simulink model "Experiment1_model"  (R2022a)
settings: Solver=FixedStepAuto  StartTime=0.0  StopTime=20  RelTol=1e-3
libraries: slpidlib x32, slctrlblks x18
(part 3 of 5)

== system Experiment1_model/Controller3 PID/controller robot7 ==
  x_rob2 : Inport
  Add : Sum
  Demux : Demux  Outputs=2
  Demux1 : Demux  Outputs=2
  Mux : Mux  Inputs=2
  PID Controller : slpidlib/PID Controller  Controller=PID  Form=Parallel  TimeDomain=Continuous-time  UseExternalTs=off  SampleTime=-1  IntegratorMethod=Forward Euler  FilterMethod=Forward Euler  ControllerParametersSource=internal  P=5  I=0  UseKiTs=off  D=0  N=100  UseFilter=on  TunerSelectOption=Transfer Function Based (PID Tuner App)  InitialConditionSource=internal  InitialConditionForIntegrator=0  InitialConditionForFilter=0  DifferentiatorICPrevScaledInput=0  ExternalReset=none  TrackingMode=off  Kt=1  LimitOutput=off  SatLimitsSource=internal  UpperSaturationLimit=inf  LowerSaturationLimit=-inf  LinearizeAsGain=on  AntiWindupMode=none  Kb=1  POutMin=[]  POutMax=[]  IOutMin=[]  IOutMax=[]  DOutMin=[]  DOutMax=[]  NOutMin=[]  NOutMax=[]  SumOutMin=[]  SumOutMax=[]  SaturationOutMin=[]  SaturationOutMax=[]  PParamMin=[]  PParamMax=[]  IParamMin=[]  IParamMax=[]  DParamMin=[]  DParamMax=[]  NParamMin=[]  NParamMax=[]  KbParamMin=[]  KbParamMax=[]  KtParamMin=[]  KtParamMax=[]  KbOutMin=[]  KbOutMax=[]  KtOutMin=[]  KtOutMax=[]  IntegratorOutMin=[]  IntegratorOutMax=[]  FilterOutMin=[]  FilterOutMax=[]  SumI1OutMin=[]  SumI1OutMax=[]  SumI2OutMin=[]  SumI2OutMax=[]  SumI3OutMin=[]  SumI3OutMax=[]  SumI4OutMin=[]  SumI4OutMax=[]  SumDOutMin=[]  SumDOutMax=[]  DifferentiatorOutMin=[]  DifferentiatorOutMax=[]  FilterDiffOutCoefMin=[]  FilterDiffOutCoefMax=[]  ReciprocalOutMin=[]  ReciprocalOutMax=[]  SumDenOutMin=[]  SumDenOutMax=[]  SumNumOutMin=[]  SumNumOutMax=[]  DivideOutMin=[]  DivideOutMax=[]  UdiffTsProdOutMin=[]  UdiffTsProdOutMax=[]  NTsProdOutMin=[]  NTsProdOutMax=[]  UintegralTsProdOutMin=[]  UintegralTsProdOutMax=[]  UngainTsProdOutMin=[]  UngainTsProdOutMax=[]  IntegratorContinuousStateAttributes=''  IntegratorStateMustResolveToSignalObject=off  IntegratorRTWStateStorageClass=Auto  FilterContinuousStateAttributes=''  FilterStateMustResolveToSignalObject=off  FilterRTWStateStorageClass=Auto  ParallelPVariant=InternalParameters  IdealPVariant=Disabled  IVariant=InternalParameters  DVariant=InternalParameters  IntegratorVariant=Continuous  SatVariant=Disabled  AWVariant=Passthrough  PCopyVariant=Disabled  TRVariant=Disabled  FdbkBlocksVariant=Forward  IdealPFdbkVariant=Disabled  SatFdbkVariant=Disabled  DerivativeFilterVariant=ContFilter  NVariant=InternalParameters  NCopyVariant=Disabled  FilterICVariant=InternalICsFilter  IntegratorICVariant=InternalICs  ExternalResetVariant=Disabled  TRSumVariant=Passthrough  SumFdbkVariant=Disabled  SumVariant=Sum_PID  TsampFilterVariant=InternalTs  TsampNgainVariant=Passthrough  TsampIntegralVariant=Passthrough  ExternalSaturationOutDataTypeStr=Inherit: Same as second input  aMode=0
  Ref_p1 : Constant  Value=[-10;10]  VectorParams1D=off
  Ref_v1 : Constant  Value=[0;0]  VectorParams1D=off
  Sum : Sum  Inputs=+-|
  Sum1 : Sum  Inputs=|-+
  u07 : Outport
  wires:
  x_rob2/1 -> Demux/1
  Demux/1 -> Sum/2
  Ref_p1/1 -> Sum/1
  Demux/2 -> Sum1/1
  Ref_v1/1 -> Sum1/2
  PID Controller/1 -> Demux1/1
  Demux1/2 -> Add/2
  Add/1 -> u07/1
  Demux1/1 -> Add/1
  Mux/1 -> PID Controller/1
  Sum1/1 -> Mux/2
  Sum/1 -> Mux/1

== system Experiment1_model/Controller3 PID/controller robot8 ==
  x_rob2 : Inport
  Add : Sum
  Demux : Demux  Outputs=2
  Demux1 : Demux  Outputs=2
  Mux : Mux  Inputs=2
  PID Controller : slpidlib/PID Controller  Controller=PID  Form=Parallel  TimeDomain=Continuous-time  UseExternalTs=off  SampleTime=-1  IntegratorMethod=Forward Euler  FilterMethod=Forward Euler  ControllerParametersSource=internal  P=5  I=0  UseKiTs=off  D=0  N=100  UseFilter=on  TunerSelectOption=Transfer Function Based (PID Tuner App)  InitialConditionSource=internal  InitialConditionForIntegrator=0  InitialConditionForFilter=0  DifferentiatorICPrevScaledInput=0  ExternalReset=none  TrackingMode=off  Kt=1  LimitOutput=off  SatLimitsSource=internal  UpperSaturationLimit=inf  LowerSaturationLimit=-inf  LinearizeAsGain=on  AntiWindupMode=none  Kb=1  POutMin=[]  POutMax=[]  IOutMin=[]  IOutMax=[]  DOutMin=[]  DOutMax=[]  NOutMin=[]  NOutMax=[]  SumOutMin=[]  SumOutMax=[]  SaturationOutMin=[]  SaturationOutMax=[]  PParamMin=[]  PParamMax=[]  IParamMin=[]  IParamMax=[]  DParamMin=[]  DParamMax=[]  NParamMin=[]  NParamMax=[]  KbParamMin=[]  KbParamMax=[]  KtParamMin=[]  KtParamMax=[]  KbOutMin=[]  KbOutMax=[]  KtOutMin=[]  KtOutMax=[]  IntegratorOutMin=[]  IntegratorOutMax=[]  FilterOutMin=[]  FilterOutMax=[]  SumI1OutMin=[]  SumI1OutMax=[]  SumI2OutMin=[]  SumI2OutMax=[]  SumI3OutMin=[]  SumI3OutMax=[]  SumI4OutMin=[]  SumI4OutMax=[]  SumDOutMin=[]  SumDOutMax=[]  DifferentiatorOutMin=[]  DifferentiatorOutMax=[]  FilterDiffOutCoefMin=[]  FilterDiffOutCoefMax=[]  ReciprocalOutMin=[]  ReciprocalOutMax=[]  SumDenOutMin=[]  SumDenOutMax=[]  SumNumOutMin=[]  SumNumOutMax=[]  DivideOutMin=[]  DivideOutMax=[]  UdiffTsProdOutMin=[]  UdiffTsProdOutMax=[]  NTsProdOutMin=[]  NTsProdOutMax=[]  UintegralTsProdOutMin=[]  UintegralTsProdOutMax=[]  UngainTsProdOutMin=[]  UngainTsProdOutMax=[]  IntegratorContinuousStateAttributes=''  IntegratorStateMustResolveToSignalObject=off  IntegratorRTWStateStorageClass=Auto  FilterContinuousStateAttributes=''  FilterStateMustResolveToSignalObject=off  FilterRTWStateStorageClass=Auto  ParallelPVariant=InternalParameters  IdealPVariant=Disabled  IVariant=InternalParameters  DVariant=InternalParameters  IntegratorVariant=Continuous  SatVariant=Disabled  AWVariant=Passthrough  PCopyVariant=Disabled  TRVariant=Disabled  FdbkBlocksVariant=Forward  IdealPFdbkVariant=Disabled  SatFdbkVariant=Disabled  DerivativeFilterVariant=ContFilter  NVariant=InternalParameters  NCopyVariant=Disabled  FilterICVariant=InternalICsFilter  IntegratorICVariant=InternalICs  ExternalResetVariant=Disabled  TRSumVariant=Passthrough  SumFdbkVariant=Disabled  SumVariant=Sum_PID  TsampFilterVariant=InternalTs  TsampNgainVariant=Passthrough  TsampIntegralVariant=Passthrough  ExternalSaturationOutDataTypeStr=Inherit: Same as second input  aMode=0
  Ref_p1 : Constant  Value=[-10;0.5]  VectorParams1D=off
  Ref_v1 : Constant  Value=[0;0]  VectorParams1D=off
  Sum : Sum  Inputs=+-|
  Sum1 : Sum  Inputs=|-+
  u08 : Outport
  wires:
  x_rob2/1 -> Demux/1
  Demux/1 -> Sum/2
  Ref_p1/1 -> Sum/1
  Demux/2 -> Sum1/1
  Ref_v1/1 -> Sum1/2
  PID Controller/1 -> Demux1/1
  Demux1/2 -> Add/2
  Add/1 -> u08/1
  Demux1/1 -> Add/1
  Mux/1 -> PID Controller/1
  Sum1/1 -> Mux/2
  Sum/1 -> Mux/1

== system Experiment1_model/Controller3 PID1/controller robot1 ==
  x_rob1 : Inport
  Add : Sum
  Demux : Demux  Outputs=2
  Demux1 : Demux  Outputs=2
  Demux2 : Demux  Outputs=2
  Mux : Mux  Inputs=2
  PID Controller : slpidlib/PID Controller  Controller=PID  Form=Parallel  TimeDomain=Continuous-time  UseExternalTs=off  SampleTime=-1  IntegratorMethod=Forward Euler  FilterMethod=Forward Euler  ControllerParametersSource=internal  P=5  I=0.0000001  UseKiTs=off  D=0.01  N=1  UseFilter=on  TunerSelectOption=Transfer Function Based (PID Tuner App)  InitialConditionSource=internal  InitialConditionForIntegrator=0  InitialConditionForFilter=0  DifferentiatorICPrevScaledInput=0  ExternalReset=none  TrackingMode=off  Kt=1  LimitOutput=off  SatLimitsSource=internal  UpperSaturationLimit=inf  LowerSaturationLimit=-inf  LinearizeAsGain=on  AntiWindupMode=none  Kb=1  POutMin=[]  POutMax=[]  IOutMin=[]  IOutMax=[]  DOutMin=[]  DOutMax=[]  NOutMin=[]  NOutMax=[]  SumOutMin=[]  SumOutMax=[]  SaturationOutMin=[]  SaturationOutMax=[]  PParamMin=[]  PParamMax=[]  IParamMin=[]  IParamMax=[]  DParamMin=[]  DParamMax=[]  NParamMin=[]  NParamMax=[]  KbParamMin=[]  KbParamMax=[]  KtParamMin=[]  KtParamMax=[]  KbOutMin=[]  KbOutMax=[]  KtOutMin=[]  KtOutMax=[]  IntegratorOutMin=[]  IntegratorOutMax=[]  FilterOutMin=[]  FilterOutMax=[]  SumI1OutMin=[]  SumI1OutMax=[]  SumI2OutMin=[]  SumI2OutMax=[]  SumI3OutMin=[]  SumI3OutMax=[]  SumI4OutMin=[]  SumI4OutMax=[]  SumDOutMin=[]  SumDOutMax=[]  DifferentiatorOutMin=[]  DifferentiatorOutMax=[]  FilterDiffOutCoefMin=[]  FilterDiffOutCoefMax=[]  ReciprocalOutMin=[]  ReciprocalOutMax=[]  SumDenOutMin=[]  SumDenOutMax=[]  SumNumOutMin=[]  SumNumOutMax=[]  DivideOutMin=[]  DivideOutMax=[]  UdiffTsProdOutMin=[]  UdiffTsProdOutMax=[]  NTsProdOutMin=[]  NTsProdOutMax=[]  UintegralTsProdOutMin=[]  UintegralTsProdOutMax=[]  UngainTsProdOutMin=[]  UngainTsProdOutMax=[]  IntegratorContinuousStateAttributes=''  IntegratorStateMustResolveToSignalObject=off  IntegratorRTWStateStorageClass=Auto  FilterContinuousStateAttributes=''  FilterStateMustResolveToSignalObject=off  FilterRTWStateStorageClass=Auto  ParallelPVariant=InternalParameters  IdealPVariant=Disabled  IVariant=InternalParameters  DVariant=InternalParameters  IntegratorVariant=Continuous  SatVariant=Disabled  AWVariant=Passthrough  PCopyVariant=Disabled  TRVariant=Disabled  FdbkBlocksVariant=Forward  IdealPFdbkVariant=Disabled  SatFdbkVariant=Disabled  DerivativeFilterVariant=ContFilter  NVariant=InternalParameters  NCopyVariant=Disabled  FilterICVariant=InternalICsFilter  IntegratorICVariant=InternalICs  ExternalResetVariant=Disabled  TRSumVariant=Passthrough  SumFdbkVariant=Disabled  SumVariant=Sum_PID  TsampFilterVariant=InternalTs  TsampNgainVariant=Passthrough  TsampIntegralVariant=Passthrough  ExternalSaturationOutDataTypeStr=Inherit: Same as second input  aMode=0
  Ref_p1 : Constant  Value=[10;0]  VectorParams1D=off
  Ref_v1 : Constant  Value=[0;0]  VectorParams1D=off
  Scope : Scope
  Scope1 : Scope
  Sum : Sum  Inputs=+-|
  Sum1 : Sum  Inputs=|-+
  Terminator : Terminator
  u01 : Outport
  wires:
  x_rob1/1 -> Demux/1
  Demux/1 -> Sum/2
  Ref_p1/1 -> Sum/1
  Demux/2 -> Sum1/1
  Ref_v1/1 -> Sum1/2
  Sum/1 -> Mux/1, Demux2/1
  Sum1/1 -> Mux/2, Scope/1
  Mux/1 -> PID Controller/1
  PID Controller/1 -> Demux1/1
  Demux1/2 -> Add/2
  Demux1/1 -> Add/1
  Add/1 -> u01/1
  Demux2/1 -> Terminator/1
  Demux2/2 -> Scope1/1

== system Experiment1_model/Controller3 PID1/controller robot2 ==
  x_rob2 : Inport
  Add : Sum
  Demux : Demux  Outputs=2
  Demux1 : Demux  Outputs=2
  Mux : Mux  Inputs=2
  PID Controller : slpidlib/PID Controller  Controller=PID  Form=Parallel  TimeDomain=Continuous-time  UseExternalTs=off  SampleTime=-1  IntegratorMethod=Forward Euler  FilterMethod=Forward Euler  ControllerParametersSource=internal  P=5  I=0.0000001  UseKiTs=off  D=0.01  N=1  UseFilter=on  TunerSelectOption=Transfer Function Based (PID Tuner App)  InitialConditionSource=internal  InitialConditionForIntegrator=0  InitialConditionForFilter=0  DifferentiatorICPrevScaledInput=0  ExternalReset=none  TrackingMode=off  Kt=1  LimitOutput=off  SatLimitsSource=internal  UpperSaturationLimit=inf  LowerSaturationLimit=-inf  LinearizeAsGain=on  AntiWindupMode=none  Kb=1  POutMin=[]  POutMax=[]  IOutMin=[]  IOutMax=[]  DOutMin=[]  DOutMax=[]  NOutMin=[]  NOutMax=[]  SumOutMin=[]  SumOutMax=[]  SaturationOutMin=[]  SaturationOutMax=[]  PParamMin=[]  PParamMax=[]  IParamMin=[]  IParamMax=[]  DParamMin=[]  DParamMax=[]  NParamMin=[]  NParamMax=[]  KbParamMin=[]  KbParamMax=[]  KtParamMin=[]  KtParamMax=[]  KbOutMin=[]  KbOutMax=[]  KtOutMin=[]  KtOutMax=[]  IntegratorOutMin=[]  IntegratorOutMax=[]  FilterOutMin=[]  FilterOutMax=[]  SumI1OutMin=[]  SumI1OutMax=[]  SumI2OutMin=[]  SumI2OutMax=[]  SumI3OutMin=[]  SumI3OutMax=[]  SumI4OutMin=[]  SumI4OutMax=[]  SumDOutMin=[]  SumDOutMax=[]  DifferentiatorOutMin=[]  DifferentiatorOutMax=[]  FilterDiffOutCoefMin=[]  FilterDiffOutCoefMax=[]  ReciprocalOutMin=[]  ReciprocalOutMax=[]  SumDenOutMin=[]  SumDenOutMax=[]  SumNumOutMin=[]  SumNumOutMax=[]  DivideOutMin=[]  DivideOutMax=[]  UdiffTsProdOutMin=[]  UdiffTsProdOutMax=[]  NTsProdOutMin=[]  NTsProdOutMax=[]  UintegralTsProdOutMin=[]  UintegralTsProdOutMax=[]  UngainTsProdOutMin=[]  UngainTsProdOutMax=[]  IntegratorContinuousStateAttributes=''  IntegratorStateMustResolveToSignalObject=off  IntegratorRTWStateStorageClass=Auto  FilterContinuousStateAttributes=''  FilterStateMustResolveToSignalObject=off  FilterRTWStateStorageClass=Auto  ParallelPVariant=InternalParameters  IdealPVariant=Disabled  IVariant=InternalParameters  DVariant=InternalParameters  IntegratorVariant=Continuous  SatVariant=Disabled  AWVariant=Passthrough  PCopyVariant=Disabled  TRVariant=Disabled  FdbkBlocksVariant=Forward  IdealPFdbkVariant=Disabled  SatFdbkVariant=Disabled  DerivativeFilterVariant=ContFilter  NVariant=InternalParameters  NCopyVariant=Disabled  FilterICVariant=InternalICsFilter  IntegratorICVariant=InternalICs  ExternalResetVariant=Disabled  TRSumVariant=Passthrough  SumFdbkVariant=Disabled  SumVariant=Sum_PID  TsampFilterVariant=InternalTs  TsampNgainVariant=Passthrough  TsampIntegralVariant=Passthrough  ExternalSaturationOutDataTypeStr=Inherit: Same as second input  aMode=0
  Ref_p1 : Constant  Value=[8;8]  VectorParams1D=off
  Ref_v1 : Constant  Value=[0;0]  VectorParams1D=off
  Scope : Scope
  Sum : Sum  Inputs=+-|
  Sum1 : Sum  Inputs=|-+
  u02 : Outport
  wires:
  x_rob2/1 -> Demux/1
  Demux/1 -> Sum/2
  Ref_p1/1 -> Sum/1
  Demux/2 -> Sum1/1
  Ref_v1/1 -> Sum1/2
  Add/1 -> u02/1
  Demux1/2 -> Add/2
  Mux/1 -> PID Controller/1
  Sum/1 -> Scope/1, Mux/1
  Sum1/1 -> Mux/2
  PID Controller/1 -> Demux1/1
  Demux1/1 -> Add/1

== system Experiment1_model/Controller3 PID1/controller robot3 ==
  x_rob2 : Inport
  Add : Sum
  Demux : Demux  Outputs=2
  Demux1 : Demux  Outputs=2
  Mux : Mux  Inputs=2
  PID Controller : slpidlib/PID Controller  Controller=PID  Form=Parallel  TimeDomain=Continuous-time  UseExternalTs=off  SampleTime=-1  IntegratorMethod=Forward Euler  FilterMethod=Forward Euler  ControllerParametersSource=internal  P=5  I=0.0000001  UseKiTs=off  D=0.01  N=1  UseFilter=on  TunerSelectOption=Transfer Function Based (PID Tuner App)  InitialConditionSource=internal  InitialConditionForIntegrator=0  InitialConditionForFilter=0  DifferentiatorICPrevScaledInput=0  ExternalReset=none  TrackingMode=off  Kt=1  LimitOutput=off  SatLimitsSource=internal  UpperSaturationLimit=inf  LowerSaturationLimit=-inf  LinearizeAsGain=on  AntiWindupMode=none  Kb=1  POutMin=[]  POutMax=[]  IOutMin=[]  IOutMax=[]  DOutMin=[]  DOutMax=[]  NOutMin=[]  NOutMax=[]  SumOutMin=[]  SumOutMax=[]  SaturationOutMin=[]  SaturationOutMax=[]  PParamMin=[]  PParamMax=[]  IParamMin=[]  IParamMax=[]  DParamMin=[]  DParamMax=[]  NParamMin=[]  NParamMax=[]  KbParamMin=[]  KbParamMax=[]  KtParamMin=[]  KtParamMax=[]  KbOutMin=[]  KbOutMax=[]  KtOutMin=[]  KtOutMax=[]  IntegratorOutMin=[]  IntegratorOutMax=[]  FilterOutMin=[]  FilterOutMax=[]  SumI1OutMin=[]  SumI1OutMax=[]  SumI2OutMin=[]  SumI2OutMax=[]  SumI3OutMin=[]  SumI3OutMax=[]  SumI4OutMin=[]  SumI4OutMax=[]  SumDOutMin=[]  SumDOutMax=[]  DifferentiatorOutMin=[]  DifferentiatorOutMax=[]  FilterDiffOutCoefMin=[]  FilterDiffOutCoefMax=[]  ReciprocalOutMin=[]  ReciprocalOutMax=[]  SumDenOutMin=[]  SumDenOutMax=[]  SumNumOutMin=[]  SumNumOutMax=[]  DivideOutMin=[]  DivideOutMax=[]  UdiffTsProdOutMin=[]  UdiffTsProdOutMax=[]  NTsProdOutMin=[]  NTsProdOutMax=[]  UintegralTsProdOutMin=[]  UintegralTsProdOutMax=[]  UngainTsProdOutMin=[]  UngainTsProdOutMax=[]  IntegratorContinuousStateAttributes=''  IntegratorStateMustResolveToSignalObject=off  IntegratorRTWStateStorageClass=Auto  FilterContinuousStateAttributes=''  FilterStateMustResolveToSignalObject=off  FilterRTWStateStorageClass=Auto  ParallelPVariant=InternalParameters  IdealPVariant=Disabled  IVariant=InternalParameters  DVariant=InternalParameters  IntegratorVariant=Continuous  SatVariant=Disabled  AWVariant=Passthrough  PCopyVariant=Disabled  TRVariant=Disabled  FdbkBlocksVariant=Forward  IdealPFdbkVariant=Disabled  SatFdbkVariant=Disabled  DerivativeFilterVariant=ContFilter  NVariant=InternalParameters  NCopyVariant=Disabled  FilterICVariant=InternalICsFilter  IntegratorICVariant=InternalICs  ExternalResetVariant=Disabled  TRSumVariant=Passthrough  SumFdbkVariant=Disabled  SumVariant=Sum_PID  TsampFilterVariant=InternalTs  TsampNgainVariant=Passthrough  TsampIntegralVariant=Passthrough  ExternalSaturationOutDataTypeStr=Inherit: Same as second input  aMode=0
  Ref_p1 : Constant  Value=[10;-10]  VectorParams1D=off
  Ref_v1 : Constant  Value=[0;0]  VectorParams1D=off
  Sum : Sum  Inputs=+-|
  Sum1 : Sum  Inputs=|-+
  u03 : Outport
  wires:
  x_rob2/1 -> Demux/1
  Demux/1 -> Sum/2
  Ref_p1/1 -> Sum/1
  Demux/2 -> Sum1/1
  Ref_v1/1 -> Sum1/2
  Add/1 -> u03/1
  Demux1/2 -> Add/2
  Demux1/1 -> Add/1
  Sum1/1 -> Mux/2
  Sum/1 -> Mux/1
  PID Controller/1 -> Demux1/1
  Mux/1 -> PID Controller/1

== system Experiment1_model/Controller3 PID1/controller robot4 ==
  x_rob2 : Inport
  Add : Sum
  Demux : Demux  Outputs=2
  Demux1 : Demux  Outputs=2
  Mux : Mux  Inputs=2
  PID Controller : slpidlib/PID Controller  Controller=PID  Form=Parallel  TimeDomain=Continuous-time  UseExternalTs=off  SampleTime=-1  IntegratorMethod=Forward Euler  FilterMethod=Forward Euler  ControllerParametersSource=internal  P=5  I=0.0000001  UseKiTs=off  D=0.01  N=1  UseFilter=on  TunerSelectOption=Transfer Function Based (PID Tuner App)  InitialConditionSource=internal  InitialConditionForIntegrator=0  InitialConditionForFilter=0  DifferentiatorICPrevScaledInput=0  ExternalReset=none  TrackingMode=off  Kt=1  LimitOutput=off  SatLimitsSource=internal  UpperSaturationLimit=inf  LowerSaturationLimit=-inf  LinearizeAsGain=on  AntiWindupMode=none  Kb=1  POutMin=[]  POutMax=[]  IOutMin=[]  IOutMax=[]  DOutMin=[]  DOutMax=[]  NOutMin=[]  NOutMax=[]  SumOutMin=[]  SumOutMax=[]  SaturationOutMin=[]  SaturationOutMax=[]  PParamMin=[]  PParamMax=[]  IParamMin=[]  IParamMax=[]  DParamMin=[]  DParamMax=[]  NParamMin=[]  NParamMax=[]  KbParamMin=[]  KbParamMax=[]  KtParamMin=[]  KtParamMax=[]  KbOutMin=[]  KbOutMax=[]  KtOutMin=[]  KtOutMax=[]  IntegratorOutMin=[]  IntegratorOutMax=[]  FilterOutMin=[]  FilterOutMax=[]  SumI1OutMin=[]  SumI1OutMax=[]  SumI2OutMin=[]  SumI2OutMax=[]  SumI3OutMin=[]  SumI3OutMax=[]  SumI4OutMin=[]  SumI4OutMax=[]  SumDOutMin=[]  SumDOutMax=[]  DifferentiatorOutMin=[]  DifferentiatorOutMax=[]  FilterDiffOutCoefMin=[]  FilterDiffOutCoefMax=[]  ReciprocalOutMin=[]  ReciprocalOutMax=[]  SumDenOutMin=[]  SumDenOutMax=[]  SumNumOutMin=[]  SumNumOutMax=[]  DivideOutMin=[]  DivideOutMax=[]  UdiffTsProdOutMin=[]  UdiffTsProdOutMax=[]  NTsProdOutMin=[]  NTsProdOutMax=[]  UintegralTsProdOutMin=[]  UintegralTsProdOutMax=[]  UngainTsProdOutMin=[]  UngainTsProdOutMax=[]  IntegratorContinuousStateAttributes=''  IntegratorStateMustResolveToSignalObject=off  IntegratorRTWStateStorageClass=Auto  FilterContinuousStateAttributes=''  FilterStateMustResolveToSignalObject=off  FilterRTWStateStorageClass=Auto  ParallelPVariant=InternalParameters  IdealPVariant=Disabled  IVariant=InternalParameters  DVariant=InternalParameters  IntegratorVariant=Continuous  SatVariant=Disabled  AWVariant=Passthrough  PCopyVariant=Disabled  TRVariant=Disabled  FdbkBlocksVariant=Forward  IdealPFdbkVariant=Disabled  SatFdbkVariant=Disabled  DerivativeFilterVariant=ContFilter  NVariant=InternalParameters  NCopyVariant=Disabled  FilterICVariant=InternalICsFilter  IntegratorICVariant=InternalICs  ExternalResetVariant=Disabled  TRSumVariant=Passthrough  SumFdbkVariant=Disabled  SumVariant=Sum_PID  TsampFilterVariant=InternalTs  TsampNgainVariant=Passthrough  TsampIntegralVariant=Passthrough  ExternalSaturationOutDataTypeStr=Inherit: Same as second input  aMode=0
  Ref_p1 : Constant  Value=[0;-10]  VectorParams1D=off
  Ref_v1 : Constant  Value=[0;0]  VectorParams1D=off
  Sum : Sum  Inputs=+-|
  Sum1 : Sum  Inputs=|-+
  u04 : Outport
  wires:
  x_rob2/1 -> Demux/1
  Demux/1 -> Sum/2
  Ref_p1/1 -> Sum/1
  Demux/2 -> Sum1/1
  Ref_v1/1 -> Sum1/2
  PID Controller/1 -> Demux1/1
  Demux1/2 -> Add/2
  Add/1 -> u04/1
  Demux1/1 -> Add/1
  Mux/1 -> PID Controller/1
  Sum1/1 -> Mux/2
  Sum/1 -> Mux/1

== system Experiment1_model/Controller3 PID1/controller robot5 ==
  x_rob2 : Inport
  Add : Sum
  Demux : Demux  Outputs=2
  Demux1 : Demux  Outputs=2
  Mux : Mux  Inputs=2
  PID Controller : slpidlib/PID Controller  Controller=PID  Form=Parallel  TimeDomain=Continuous-time  UseExternalTs=off  SampleTime=-1  IntegratorMethod=Forward Euler  FilterMethod=Forward Euler  ControllerParametersSource=internal  P=5  I=0  UseKiTs=off  D=0  N=100  UseFilter=on  TunerSelectOption=Transfer Function Based (PID Tuner App)  InitialConditionSource=internal  InitialConditionForIntegrator=0  InitialConditionForFilter=0  DifferentiatorICPrevScaledInput=0  ExternalReset=none  TrackingMode=off  Kt=1  LimitOutput=off  SatLimitsSource=internal  UpperSaturationLimit=inf  LowerSaturationLimit=-inf  LinearizeAsGain=on  AntiWindupMode=none  Kb=1  POutMin=[]  POutMax=[]  IOutMin=[]  IOutMax=[]  DOutMin=[]  DOutMax=[]  NOutMin=[]  NOutMax=[]  SumOutMin=[]  SumOutMax=[]  SaturationOutMin=[]  SaturationOutMax=[]  PParamMin=[]  PParamMax=[]  IParamMin=[]  IParamMax=[]  DParamMin=[]  DParamMax=[]  NParamMin=[]  NParamMax=[]  KbParamMin=[]  KbParamMax=[]  KtParamMin=[]  KtParamMax=[]  KbOutMin=[]  KbOutMax=[]  KtOutMin=[]  KtOutMax=[]  IntegratorOutMin=[]  IntegratorOutMax=[]  FilterOutMin=[]  FilterOutMax=[]  SumI1OutMin=[]  SumI1OutMax=[]  SumI2OutMin=[]  SumI2OutMax=[]  SumI3OutMin=[]  SumI3OutMax=[]  SumI4OutMin=[]  SumI4OutMax=[]  SumDOutMin=[]  SumDOutMax=[]  DifferentiatorOutMin=[]  DifferentiatorOutMax=[]  FilterDiffOutCoefMin=[]  FilterDiffOutCoefMax=[]  ReciprocalOutMin=[]  ReciprocalOutMax=[]  SumDenOutMin=[]  SumDenOutMax=[]  SumNumOutMin=[]  SumNumOutMax=[]  DivideOutMin=[]  DivideOutMax=[]  UdiffTsProdOutMin=[]  UdiffTsProdOutMax=[]  NTsProdOutMin=[]  NTsProdOutMax=[]  UintegralTsProdOutMin=[]  UintegralTsProdOutMax=[]  UngainTsProdOutMin=[]  UngainTsProdOutMax=[]  IntegratorContinuousStateAttributes=''  IntegratorStateMustResolveToSignalObject=off  IntegratorRTWStateStorageClass=Auto  FilterContinuousStateAttributes=''  FilterStateMustResolveToSignalObject=off  FilterRTWStateStorageClass=Auto  ParallelPVariant=InternalParameters  IdealPVariant=Disabled  IVariant=InternalParameters  DVariant=InternalParameters  IntegratorVariant=Continuous  SatVariant=Disabled  AWVariant=Passthrough  PCopyVariant=Disabled  TRVariant=Disabled  FdbkBlocksVariant=Forward  IdealPFdbkVariant=Disabled  SatFdbkVariant=Disabled  DerivativeFilterVariant=ContFilter  NVariant=InternalParameters  NCopyVariant=Disabled  FilterICVariant=InternalICsFilter  IntegratorICVariant=InternalICs  ExternalResetVariant=Disabled  TRSumVariant=Passthrough  SumFdbkVariant=Disabled  SumVariant=Sum_PID  TsampFilterVariant=InternalTs  TsampNgainVariant=Passthrough  TsampIntegralVariant=Passthrough  ExternalSaturationOutDataTypeStr=Inherit: Same as second input  aMode=0
  Ref_p1 : Constant  Value=[0;10]  VectorParams1D=off
  Ref_v1 : Constant  Value=[0;0]  VectorParams1D=off
  Sum : Sum  Inputs=+-|
  Sum1 : Sum  Inputs=|-+
  u05 : Outport
  wires:
  x_rob2/1 -> Demux/1
  Demux/1 -> Sum/2
  Ref_p1/1 -> Sum/1
  Demux/2 -> Sum1/1
  Ref_v1/1 -> Sum1/2
  Add/1 -> u05/1
  PID Controller/1 -> Demux1/1
  Demux1/2 -> Add/2
  Demux1/1 -> Add/1
  Mux/1 -> PID Controller/1
  Sum1/1 -> Mux/2
  Sum/1 -> Mux/1

== system Experiment1_model/Controller3 PID1/controller robot6 ==
  x_rob2 : Inport
  Add : Sum
  Demux : Demux  Outputs=2
  Demux1 : Demux  Outputs=2
  Mux : Mux  Inputs=2
  PID Controller : slpidlib/PID Controller  Controller=PID  Form=Parallel  TimeDomain=Continuous-time  UseExternalTs=off  SampleTime=-1  IntegratorMethod=Forward Euler  FilterMethod=Forward Euler  ControllerParametersSource=internal  P=5  I=0  UseKiTs=off  D=0  N=100  UseFilter=on  TunerSelectOption=Transfer Function Based (PID Tuner App)  InitialConditionSource=internal  InitialConditionForIntegrator=0  InitialConditionForFilter=0  DifferentiatorICPrevScaledInput=0  ExternalReset=none  TrackingMode=off  Kt=1  LimitOutput=off  SatLimitsSource=internal  UpperSaturationLimit=inf  LowerSaturationLimit=-inf  LinearizeAsGain=on  AntiWindupMode=none  Kb=1  POutMin=[]  POutMax=[]  IOutMin=[]  IOutMax=[]  DOutMin=[]  DOutMax=[]  NOutMin=[]  NOutMax=[]  SumOutMin=[]  SumOutMax=[]  SaturationOutMin=[]  SaturationOutMax=[]  PParamMin=[]  PParamMax=[]  IParamMin=[]  IParamMax=[]  DParamMin=[]  DParamMax=[]  NParamMin=[]  NParamMax=[]  KbParamMin=[]  KbParamMax=[]  KtParamMin=[]  KtParamMax=[]  KbOutMin=[]  KbOutMax=[]  KtOutMin=[]  KtOutMax=[]  IntegratorOutMin=[]  IntegratorOutMax=[]  FilterOutMin=[]  FilterOutMax=[]  SumI1OutMin=[]  SumI1OutMax=[]  SumI2OutMin=[]  SumI2OutMax=[]  SumI3OutMin=[]  SumI3OutMax=[]  SumI4OutMin=[]  SumI4OutMax=[]  SumDOutMin=[]  SumDOutMax=[]  DifferentiatorOutMin=[]  DifferentiatorOutMax=[]  FilterDiffOutCoefMin=[]  FilterDiffOutCoefMax=[]  ReciprocalOutMin=[]  ReciprocalOutMax=[]  SumDenOutMin=[]  SumDenOutMax=[]  SumNumOutMin=[]  SumNumOutMax=[]  DivideOutMin=[]  DivideOutMax=[]  UdiffTsProdOutMin=[]  UdiffTsProdOutMax=[]  NTsProdOutMin=[]  NTsProdOutMax=[]  UintegralTsProdOutMin=[]  UintegralTsProdOutMax=[]  UngainTsProdOutMin=[]  UngainTsProdOutMax=[]  IntegratorContinuousStateAttributes=''  IntegratorStateMustResolveToSignalObject=off  IntegratorRTWStateStorageClass=Auto  FilterContinuousStateAttributes=''  FilterStateMustResolveToSignalObject=off  FilterRTWStateStorageClass=Auto  ParallelPVariant=InternalParameters  IdealPVariant=Disabled  IVariant=InternalParameters  DVariant=InternalParameters  IntegratorVariant=Continuous  SatVariant=Disabled  AWVariant=Passthrough  PCopyVariant=Disabled  TRVariant=Disabled  FdbkBlocksVariant=Forward  IdealPFdbkVariant=Disabled  SatFdbkVariant=Disabled  DerivativeFilterVariant=ContFilter  NVariant=InternalParameters  NCopyVariant=Disabled  FilterICVariant=InternalICsFilter  IntegratorICVariant=InternalICs  ExternalResetVariant=Disabled  TRSumVariant=Passthrough  SumFdbkVariant=Disabled  SumVariant=Sum_PID  TsampFilterVariant=InternalTs  TsampNgainVariant=Passthrough  TsampIntegralVariant=Passthrough  ExternalSaturationOutDataTypeStr=Inherit: Same as second input  aMode=0
  Ref_p1 : Constant  Value=[-12;-6]  VectorParams1D=off
  Ref_v1 : Constant  Value=[0;0]  VectorParams1D=off
  Sum : Sum  Inputs=+-|
  Sum1 : Sum  Inputs=|-+
  u06 : Outport
  wires:
  x_rob2/1 -> Demux/1
  Demux/1 -> Sum/2
  Ref_p1/1 -> Sum/1
  Demux/2 -> Sum1/1
  Ref_v1/1 -> Sum1/2
  PID Controller/1 -> Demux1/1
  Demux1/2 -> Add/2
  Add/1 -> u06/1
  Demux1/1 -> Add/1
  Mux/1 -> PID Controller/1
  Sum1/1 -> Mux/2
  Sum/1 -> Mux/1

== system Experiment1_model/Controller3 PID1/controller robot7 ==
  x_rob2 : Inport
  Add : Sum
  Demux : Demux  Outputs=2
  Demux1 : Demux  Outputs=2
  Mux : Mux  Inputs=2
  PID Controller : slpidlib/PID Controller  Controller=PID  Form=Parallel  TimeDomain=Continuous-time  UseExternalTs=off  SampleTime=-1  IntegratorMethod=Forward Euler  FilterMethod=Forward Euler  ControllerParametersSource=internal  P=5  I=0  UseKiTs=off  D=0  N=100  UseFilter=on  TunerSelectOption=Transfer Function Based (PID Tuner App)  InitialConditionSource=internal  InitialConditionForIntegrator=0  InitialConditionForFilter=0  DifferentiatorICPrevScaledInput=0  ExternalReset=none  TrackingMode=off  Kt=1  LimitOutput=off  SatLimitsSource=internal  UpperSaturationLimit=inf  LowerSaturationLimit=-inf  LinearizeAsGain=on  AntiWindupMode=none  Kb=1  POutMin=[]  POutMax=[]  IOutMin=[]  IOutMax=[]  DOutMin=[]  DOutMax=[]  NOutMin=[]  NOutMax=[]  SumOutMin=[]  SumOutMax=[]  SaturationOutMin=[]  SaturationOutMax=[]  PParamMin=[]  PParamMax=[]  IParamMin=[]  IParamMax=[]  DParamMin=[]  DParamMax=[]  NParamMin=[]  NParamMax=[]  KbParamMin=[]  KbParamMax=[]  KtParamMin=[]  KtParamMax=[]  KbOutMin=[]  KbOutMax=[]  KtOutMin=[]  KtOutMax=[]  IntegratorOutMin=[]  IntegratorOutMax=[]  FilterOutMin=[]  FilterOutMax=[]  SumI1OutMin=[]  SumI1OutMax=[]  SumI2OutMin=[]  SumI2OutMax=[]  SumI3OutMin=[]  SumI3OutMax=[]  SumI4OutMin=[]  SumI4OutMax=[]  SumDOutMin=[]  SumDOutMax=[]  DifferentiatorOutMin=[]  DifferentiatorOutMax=[]  FilterDiffOutCoefMin=[]  FilterDiffOutCoefMax=[]  ReciprocalOutMin=[]  ReciprocalOutMax=[]  SumDenOutMin=[]  SumDenOutMax=[]  SumNumOutMin=[]  SumNumOutMax=[]  DivideOutMin=[]  DivideOutMax=[]  UdiffTsProdOutMin=[]  UdiffTsProdOutMax=[]  NTsProdOutMin=[]  NTsProdOutMax=[]  UintegralTsProdOutMin=[]  UintegralTsProdOutMax=[]  UngainTsProdOutMin=[]  UngainTsProdOutMax=[]  IntegratorContinuousStateAttributes=''  IntegratorStateMustResolveToSignalObject=off  IntegratorRTWStateStorageClass=Auto  FilterContinuousStateAttributes=''  FilterStateMustResolveToSignalObject=off  FilterRTWStateStorageClass=Auto  ParallelPVariant=InternalParameters  IdealPVariant=Disabled  IVariant=InternalParameters  DVariant=InternalParameters  IntegratorVariant=Continuous  SatVariant=Disabled  AWVariant=Passthrough  PCopyVariant=Disabled  TRVariant=Disabled  FdbkBlocksVariant=Forward  IdealPFdbkVariant=Disabled  SatFdbkVariant=Disabled  DerivativeFilterVariant=ContFilter  NVariant=InternalParameters  NCopyVariant=Disabled  FilterICVariant=InternalICsFilter  IntegratorICVariant=InternalICs  ExternalResetVariant=Disabled  TRSumVariant=Passthrough  SumFdbkVariant=Disabled  SumVariant=Sum_PID  TsampFilterVariant=InternalTs  TsampNgainVariant=Passthrough  TsampIntegralVariant=Passthrough  ExternalSaturationOutDataTypeStr=Inherit: Same as second input  aMode=0
  Ref_p1 : Constant  Value=[-10;10]  VectorParams1D=off
  Ref_v1 : Constant  Value=[0;0]  VectorParams1D=off
  Sum : Sum  Inputs=+-|
  Sum1 : Sum  Inputs=|-+
  u07 : Outport
  wires:
  x_rob2/1 -> Demux/1
  Demux/1 -> Sum/2
  Ref_p1/1 -> Sum/1
  Demux/2 -> Sum1/1
  Ref_v1/1 -> Sum1/2
  PID Controller/1 -> Demux1/1
  Demux1/2 -> Add/2
  Add/1 -> u07/1
  Demux1/1 -> Add/1
  Mux/1 -> PID Controller/1
  Sum1/1 -> Mux/2
  Sum/1 -> Mux/1

== system Experiment1_model/Controller3 PID1/controller robot8 ==
  x_rob2 : Inport
  Add : Sum
  Demux : Demux  Outputs=2
  Demux1 : Demux  Outputs=2
  Mux : Mux  Inputs=2
  PID Controller : slpidlib/PID Controller  Controller=PID  Form=Parallel  TimeDomain=Continuous-time  UseExternalTs=off  SampleTime=-1  IntegratorMethod=Forward Euler  FilterMethod=Forward Euler  ControllerParametersSource=internal  P=5  I=0  UseKiTs=off  D=0  N=100  UseFilter=on  TunerSelectOption=Transfer Function Based (PID Tuner App)  InitialConditionSource=internal  InitialConditionForIntegrator=0  InitialConditionForFilter=0  DifferentiatorICPrevScaledInput=0  ExternalReset=none  TrackingMode=off  Kt=1  LimitOutput=off  SatLimitsSource=internal  UpperSaturationLimit=inf  LowerSaturationLimit=-inf  LinearizeAsGain=on  AntiWindupMode=none  Kb=1  POutMin=[]  POutMax=[]  IOutMin=[]  IOutMax=[]  DOutMin=[]  DOutMax=[]  NOutMin=[]  NOutMax=[]  SumOutMin=[]  SumOutMax=[]  SaturationOutMin=[]  SaturationOutMax=[]  PParamMin=[]  PParamMax=[]  IParamMin=[]  IParamMax=[]  DParamMin=[]  DParamMax=[]  NParamMin=[]  NParamMax=[]  KbParamMin=[]  KbParamMax=[]  KtParamMin=[]  KtParamMax=[]  KbOutMin=[]  KbOutMax=[]  KtOutMin=[]  KtOutMax=[]  IntegratorOutMin=[]  IntegratorOutMax=[]  FilterOutMin=[]  FilterOutMax=[]  SumI1OutMin=[]  SumI1OutMax=[]  SumI2OutMin=[]  SumI2OutMax=[]  SumI3OutMin=[]  SumI3OutMax=[]  SumI4OutMin=[]  SumI4OutMax=[]  SumDOutMin=[]  SumDOutMax=[]  DifferentiatorOutMin=[]  DifferentiatorOutMax=[]  FilterDiffOutCoefMin=[]  FilterDiffOutCoefMax=[]  ReciprocalOutMin=[]  ReciprocalOutMax=[]  SumDenOutMin=[]  SumDenOutMax=[]  SumNumOutMin=[]  SumNumOutMax=[]  DivideOutMin=[]  DivideOutMax=[]  UdiffTsProdOutMin=[]  UdiffTsProdOutMax=[]  NTsProdOutMin=[]  NTsProdOutMax=[]  UintegralTsProdOutMin=[]  UintegralTsProdOutMax=[]  UngainTsProdOutMin=[]  UngainTsProdOutMax=[]  IntegratorContinuousStateAttributes=''  IntegratorStateMustResolveToSignalObject=off  IntegratorRTWStateStorageClass=Auto  FilterContinuousStateAttributes=''  FilterStateMustResolveToSignalObject=off  FilterRTWStateStorageClass=Auto  ParallelPVariant=InternalParameters  IdealPVariant=Disabled  IVariant=InternalParameters  DVariant=InternalParameters  IntegratorVariant=Continuous  SatVariant=Disabled  AWVariant=Passthrough  PCopyVariant=Disabled  TRVariant=Disabled  FdbkBlocksVariant=Forward  IdealPFdbkVariant=Disabled  SatFdbkVariant=Disabled  DerivativeFilterVariant=ContFilter  NVariant=InternalParameters  NCopyVariant=Disabled  FilterICVariant=InternalICsFilter  IntegratorICVariant=InternalICs  ExternalResetVariant=Disabled  TRSumVariant=Passthrough  SumFdbkVariant=Disabled  SumVariant=Sum_PID  TsampFilterVariant=InternalTs  TsampNgainVariant=Passthrough  TsampIntegralVariant=Passthrough  ExternalSaturationOutDataTypeStr=Inherit: Same as second input  aMode=0
  Ref_p1 : Constant  Value=[-10;0.5]  VectorParams1D=off
  Ref_v1 : Constant  Value=[0;0]  VectorParams1D=off
  Sum : Sum  Inputs=+-|
  Sum1 : Sum  Inputs=|-+
  u08 : Outport
  wires:
  x_rob2/1 -> Demux/1
  Demux/1 -> Sum/2
  Ref_p1/1 -> Sum/1
  Demux/2 -> Sum1/1
  Ref_v1/1 -> Sum1/2
  PID Controller/1 -> Demux1/1
  Demux1/2 -> Add/2
  Add/1 -> u08/1
  Demux1/1 -> Add/1
  Mux/1 -> PID Controller/1
  Sum1/1 -> Mux/2
  Sum/1 -> Mux/1

== system Experiment1_model/Robot Dynamics Centralized /Robot1 ==
  In1 : Inport
  Demux : Demux  Outputs=2
  Integrator : Integrator  InitialConditionSource=external  LimitOutput=on  UpperSaturationLimit=2  LowerSaturationLimit=-2
  Integrator1 : Integrator  InitialConditionSource=external
  initial conditions : Constant  Value=[0;0;-10;0]  VectorParams1D=off
  p1 : Outport
  v1 : Outport  Port=2
  wires:
  initial conditions/1 -> Demux/1
  In1/1 -> Integrator/1  "u1"
  Demux/1 -> Integrator/2  "v0"
  Integrator/1 -> Integrator1/1, v1/1  "v"
  Demux/2 -> Integrator1/2  "p0"
  Integrator1/1 -> p1/1  "p"

== system Experiment1_model/Robot Dynamics Centralized /Robot2 ==
  In1 : Inport
  Demux : Demux  Outputs=2
  Integrator : Integrator  InitialConditionSource=external  LimitOutput=on  UpperSaturationLimit=2  LowerSaturationLimit=-2
  Integrator1 : Integrator  InitialConditionSource=external
  initial conditions : Constant  Value=[0;0;-10;-10]  VectorParams1D=off
  p2 : Outport
  v2 : Outport  Port=2
  wires:
  initial conditions/1 -> Demux/1
  In1/1 -> Integrator/1  "u1"
  Demux/1 -> Integrator/2  "v0"
  Integrator/1 -> v2/1, Integrator1/1  "v"
  Demux/2 -> Integrator1/2  "p0"
  Integrator1/1 -> p2/1  "p"

== system Experiment1_model/Robot Dynamics Centralized /Robot3 ==
  In1 : Inport
  Demux : Demux  Outputs=2
  Integrator : Integrator  InitialConditionSource=external  LimitOutput=on  UpperSaturationLimit=2  LowerSaturationLimit=-2
  Integrator1 : Integrator  InitialConditionSource=external
  initial conditions : Constant  Value=[0;0;-10;10]  VectorParams1D=off
  p3 : Outport
  v3 : Outport  Port=2
  wires:
  initial conditions/1 -> Demux/1
  In1/1 -> Integrator/1  "u1"
  Demux/1 -> Integrator/2  "v0"
  Integrator/1 -> v3/1, Integrator1/1  "v"
  Demux/2 -> Integrator1/2  "p0"
  Integrator1/1 -> p3/1  "p"

== system Experiment1_model/Robot Dynamics Centralized /Robot4 ==
  In1 : Inport
  Demux : Demux  Outputs=2
  Integrator : Integrator  InitialConditionSource=external  LimitOutput=on  UpperSaturationLimit=2  LowerSaturationLimit=-2
  Integrator1 : Integrator  InitialConditionSource=external
  initial conditions : Constant  Value=[0;0;0;10]  VectorParams1D=off
  p4 : Outport
  v4 : Outport  Port=2
  wires:
  initial conditions/1 -> Demux/1
  In1/1 -> Integrator/1  "u1"
  Demux/1 -> Integrator/2  "v0"
  Integrator/1 -> v4/1, Integrator1/1  "v"
  Demux/2 -> Integrator1/2  "p0"
  Integrator1/1 -> p4/1  "p"

== system Experiment1_model/Robot Dynamics Centralized /Robot5 ==
  In1 : Inport
  Demux : Demux  Outputs=2
  Integrator : Integrator  InitialConditionSource=external  LimitOutput=on  UpperSaturationLimit=2  LowerSaturationLimit=-2
  Integrator1 : Integrator  InitialConditionSource=external
  initial conditions : Constant  Value=[0;0;-1;-10]  VectorParams1D=off
  p5 : Outport
  v5 : Outport  Port=2
  wires:
  initial conditions/1 -> Demux/1
  In1/1 -> Integrator/1  "u1"
  Demux/1 -> Integrator/2  "v0"
  Integrator/1 -> v5/1, Integrator1/1  "v"
  Demux/2 -> Integrator1/2  "p0"
  Integrator1/1 -> p5/1  "p"

== system Experiment1_model/Robot Dynamics Centralized /Robot6 ==
  In1 : Inport
  Demux : Demux  Outputs=2
  Integrator : Integrator  InitialConditionSource=external  LimitOutput=on  UpperSaturationLimit=2  LowerSaturationLimit=-2
  Integrator1 : Integrator  InitialConditionSource=external
  initial conditions : Constant  Value=[0;0;8;8]  VectorParams1D=off
  p6 : Outport
  v6 : Outport  Port=2
  wires:
  initial conditions/1 -> Demux/1
  In1/1 -> Integrator/1  "u1"
  Demux/1 -> Integrator/2  "v0"
  Integrator/1 -> v6/1, Integrator1/1  "v"
  Demux/2 -> Integrator1/2  "p0"
  Integrator1/1 -> p6/1  "p"

== system Experiment1_model/Robot Dynamics Centralized /Robot7 ==
  In1 : Inport
  Demux : Demux  Outputs=2
  Integrator : Integrator  InitialConditionSource=external  LimitOutput=on  UpperSaturationLimit=2  LowerSaturationLimit=-2
  Integrator1 : Integrator  InitialConditionSource=external
  initial conditions : Constant  Value=[0;0;10;-10]  VectorParams1D=off
  p7 : Outport
  v7 : Outport  Port=2
  wires:
  initial conditions/1 -> Demux/1
  In1/1 -> Integrator/1  "u1"
  Demux/1 -> Integrator/2  "v0"
  Integrator/1 -> v7/1, Integrator1/1  "v"
  Demux/2 -> Integrator1/2  "p0"
  Integrator1/1 -> p7/1  "p"

== system Experiment1_model/Robot Dynamics Centralized /Robot8 ==
  In1 : Inport
  Demux : Demux  Outputs=2
  Integrator : Integrator  InitialConditionSource=external  LimitOutput=on  UpperSaturationLimit=2  LowerSaturationLimit=-2
  Integrator1 : Integrator  InitialConditionSource=external
  initial conditions : Constant  Value=[0;0;12;-3]  VectorParams1D=off
  p8 : Outport
  v8 : Outport  Port=2
  wires:
  initial conditions/1 -> Demux/1
  In1/1 -> Integrator/1  "u1"
  Demux/1 -> Integrator/2  "v0"
  Integrator/1 -> v8/1, Integrator1/1  "v"
  Demux/2 -> Integrator1/2  "p0"
  Integrator1/1 -> p8/1  "p"

== system Experiment1_model/Robot Dynamics Centralized /Visualization ==
  p : Inport
  MATLAB Function : MATLAB Function  TreatAsAtomicUnit=on
  wires:
  p/1 -> MATLAB Function/1(p)

== system Experiment1_model/Robot Dynamics Centralized /Visualization1 ==
  p : Inport
  MATLAB Function : MATLAB Function  TreatAsAtomicUnit=on
  wires:
  p/1 -> MATLAB Function/1(p)

== system Experiment1_model/Robot Dynamics Centralized with Neighbours/Robot1 ==
  In1 : Inport
  Demux : Demux  Outputs=2
  Integrator : Integrator  InitialConditionSource=external  LimitOutput=on  UpperSaturationLimit=2  LowerSaturationLimit=-2
  Integrator1 : Integrator  InitialConditionSource=external
  initial conditions : Constant  Value=[0;0;-10;0]  VectorParams1D=off
  p1 : Outport
  v1 : Outport  Port=2
  wires:
  initial conditions/1 -> Demux/1
  In1/1 -> Integrator/1  "u1"
  Demux/1 -> Integrator/2  "v0"
  Integrator/1 -> Integrator1/1, v1/1  "v"
  Demux/2 -> Integrator1/2  "p0"
  Integrator1/1 -> p1/1  "p"

== system Experiment1_model/Robot Dynamics Centralized with Neighbours/Robot2 ==
  In1 : Inport
  Demux : Demux  Outputs=2
  Integrator : Integrator  InitialConditionSource=external  LimitOutput=on  UpperSaturationLimit=2  LowerSaturationLimit=-2
  Integrator1 : Integrator  InitialConditionSource=external
  initial conditions : Constant  Value=[0;0;-10;-10]  VectorParams1D=off
  p2 : Outport
  v2 : Outport  Port=2
  wires:
  initial conditions/1 -> Demux/1
  In1/1 -> Integrator/1  "u1"
  Demux/1 -> Integrator/2  "v0"
  Integrator/1 -> v2/1, Integrator1/1  "v"
  Demux/2 -> Integrator1/2  "p0"
  Integrator1/1 -> p2/1  "p"

== system Experiment1_model/Robot Dynamics Centralized with Neighbours/Robot3 ==
  In1 : Inport
  Demux : Demux  Outputs=2
  Integrator : Integrator  InitialConditionSource=external  LimitOutput=on  UpperSaturationLimit=2  LowerSaturationLimit=-2
  Integrator1 : Integrator  InitialConditionSource=external
  initial conditions : Constant  Value=[0;0;-10;10]  VectorParams1D=off
  p3 : Outport
  v3 : Outport  Port=2
  wires:
  initial conditions/1 -> Demux/1
  In1/1 -> Integrator/1  "u1"
  Demux/1 -> Integrator/2  "v0"
  Integrator/1 -> v3/1, Integrator1/1  "v"
  Demux/2 -> Integrator1/2  "p0"
  Integrator1/1 -> p3/1  "p"

== system Experiment1_model/Robot Dynamics Centralized with Neighbours/Robot4 ==
  In1 : Inport
  Demux : Demux  Outputs=2
  Integrator : Integrator  InitialConditionSource=external  LimitOutput=on  UpperSaturationLimit=2  LowerSaturationLimit=-2
  Integrator1 : Integrator  InitialConditionSource=external
  initial conditions : Constant  Value=[0;0;0;10]  VectorParams1D=off
  p4 : Outport
  v4 : Outport  Port=2
  wires:
  initial conditions/1 -> Demux/1
  In1/1 -> Integrator/1  "u1"
  Demux/1 -> Integrator/2  "v0"
  Integrator/1 -> v4/1, Integrator1/1  "v"
  Demux/2 -> Integrator1/2  "p0"
  Integrator1/1 -> p4/1  "p"

== system Experiment1_model/Robot Dynamics Centralized with Neighbours/Robot5 ==
  In1 : Inport
  Demux : Demux  Outputs=2
  Integrator : Integrator  InitialConditionSource=external  LimitOutput=on  UpperSaturationLimit=2  LowerSaturationLimit=-2
  Integrator1 : Integrator  InitialConditionSource=external
  initial conditions : Constant  Value=[0;0;-1;-10]  VectorParams1D=off
  p5 : Outport
  v5 : Outport  Port=2
  wires:
  initial conditions/1 -> Demux/1
  In1/1 -> Integrator/1  "u1"
  Demux/1 -> Integrator/2  "v0"
  Integrator/1 -> v5/1, Integrator1/1  "v"
  Demux/2 -> Integrator1/2  "p0"
  Integrator1/1 -> p5/1  "p"

== system Experiment1_model/Robot Dynamics Centralized with Neighbours/Robot6 ==
  In1 : Inport
  Demux : Demux  Outputs=2
  Integrator : Integrator  InitialConditionSource=external  LimitOutput=on  UpperSaturationLimit=2  LowerSaturationLimit=-2
  Integrator1 : Integrator  InitialConditionSource=external
  initial conditions : Constant  Value=[0;0;8;8]  VectorParams1D=off
  p6 : Outport
  v6 : Outport  Port=2
  wires:
  initial conditions/1 -> Demux/1
  In1/1 -> Integrator/1  "u1"
  Demux/1 -> Integrator/2  "v0"
  Integrator/1 -> v6/1, Integrator1/1  "v"
  Demux/2 -> Integrator1/2  "p0"
  Integrator1/1 -> p6/1  "p"

== system Experiment1_model/Robot Dynamics Centralized with Neighbours/Robot7 ==
  In1 : Inport
  Demux : Demux  Outputs=2
  Integrator : Integrator  InitialConditionSource=external  LimitOutput=on  UpperSaturationLimit=2  LowerSaturationLimit=-2
  Integrator1 : Integrator  InitialConditionSource=external
  initial conditions : Constant  Value=[0;0;10;-10]  VectorParams1D=off
  p7 : Outport
  v7 : Outport  Port=2
  wires:
  initial conditions/1 -> Demux/1
  In1/1 -> Integrator/1  "u1"
  Demux/1 -> Integrator/2  "v0"
  Integrator/1 -> v7/1, Integrator1/1  "v"
  Demux/2 -> Integrator1/2  "p0"
  Integrator1/1 -> p7/1  "p"

== system Experiment1_model/Robot Dynamics Centralized with Neighbours/Robot8 ==
  In1 : Inport
  Demux : Demux  Outputs=2
  Integrator : Integrator  InitialConditionSource=external  LimitOutput=on  UpperSaturationLimit=2  LowerSaturationLimit=-2
  Integrator1 : Integrator  InitialConditionSource=external
  initial conditions : Constant  Value=[0;0;12;-3]  VectorParams1D=off
  p8 : Outport
  v8 : Outport  Port=2
  wires:
  initial conditions/1 -> Demux/1
  In1/1 -> Integrator/1  "u1"
  Demux/1 -> Integrator/2  "v0"
  Integrator/1 -> v8/1, Integrator1/1  "v"
  Demux/2 -> Integrator1/2  "p0"
  Integrator1/1 -> p8/1  "p"

== system Experiment1_model/Robot Dynamics Centralized with Neighbours/Visualization ==
  p : Inport
  MATLAB Function : MATLAB Function  TreatAsAtomicUnit=on
  wires:
  p/1 -> MATLAB Function/1(p)

== system Experiment1_model/Robot Dynamics Centralized with Neighbours/Visualization1 ==
  p : Inport
  MATLAB Function : MATLAB Function  TreatAsAtomicUnit=on
  wires:
  p/1 -> MATLAB Function/1(p)

== system Experiment1_model/Robots Dynamics Decentralized/Robot1 ==
  In1 : Inport
  Demux : Demux  Outputs=2
  Integrator : Integrator  InitialConditionSource=external  LimitOutput=on  UpperSaturationLimit=2  LowerSaturationLimit=-2
  Integrator1 : Integrator  InitialConditionSource=external
  initial conditions : Constant  Value=[0;0;-10;0]  VectorParams1D=off
  p1 : Outport
  v1 : Outport  Port=2
  wires:
  initial conditions/1 -> Demux/1
  In1/1 -> Integrator/1  "u1"
  Demux/1 -> Integrator/2  "v0"
  Integrator/1 -> Integrator1/1, v1/1  "v"
  Demux/2 -> Integrator1/2  "p0"
  Integrator1/1 -> p1/1  "p"

== system Experiment1_model/Robots Dynamics Decentralized/Robot2 ==
  In1 : Inport
  Demux : Demux  Outputs=2
  Integrator : Integrator  InitialConditionSource=external  LimitOutput=on  UpperSaturationLimit=2  LowerSaturationLimit=-2
  Integrator1 : Integrator  InitialConditionSource=external
  initial conditions : Constant  Value=[0;0;-10;-10]  VectorParams1D=off
  p2 : Outport
  v2 : Outport  Port=2
  wires:
  initial conditions/1 -> Demux/1
  In1/1 -> Integrator/1  "u1"
  Demux/1 -> Integrator/2  "v0"
  Integrator/1 -> v2/1, Integrator1/1  "v"
  Demux/2 -> Integrator1/2  "p0"
  Integrator1/1 -> p2/1  "p"

== system Experiment1_model/Robots Dynamics Decentralized/Robot3 ==
  In1 : Inport
  Demux : Demux  Outputs=2
  Integrator : Integrator  InitialConditionSource=external  LimitOutput=on  UpperSaturationLimit=2  LowerSaturationLimit=-2
  Integrator1 : Integrator  InitialConditionSource=external
  initial conditions : Constant  Value=[0;0;-10;10]  VectorParams1D=off
  p3 : Outport
  v3 : Outport  Port=2
  wires:
  initial conditions/1 -> Demux/1
  In1/1 -> Integrator/1  "u1"
  Demux/1 -> Integrator/2  "v0"
  Integrator/1 -> v3/1, Integrator1/1  "v"
  Demux/2 -> Integrator1/2  "p0"
  Integrator1/1 -> p3/1  "p"

== system Experiment1_model/Robots Dynamics Decentralized/Robot4 ==
  In1 : Inport
  Demux : Demux  Outputs=2
  Integrator : Integrator  InitialConditionSource=external  LimitOutput=on  UpperSaturationLimit=2  LowerSaturationLimit=-2
  Integrator1 : Integrator  InitialConditionSource=external
  initial conditions : Constant  Value=[0;0;0;10]  VectorParams1D=off
  p4 : Outport
  v4 : Outport  Port=2
  wires:
  initial conditions/1 -> Demux/1
  In1/1 -> Integrator/1  "u1"
  Demux/1 -> Integrator/2  "v0"
  Integrator/1 -> v4/1, Integrator1/1  "v"
  Demux/2 -> Integrator1/2  "p0"
  Integrator1/1 -> p4/1  "p"

== system Experiment1_model/Robots Dynamics Decentralized/Robot5 ==
  In1 : Inport
  Demux : Demux  Outputs=2
  Integrator : Integrator  InitialConditionSource=external  LimitOutput=on  UpperSaturationLimit=2  LowerSaturationLimit=-2
  Integrator1 : Integrator  InitialConditionSource=external
  initial conditions : Constant  Value=[0;0;-1;-10]  VectorParams1D=off
  p5 : Outport
  v5 : Outport  Port=2
  wires:
  initial conditions/1 -> Demux/1
  In1/1 -> Integrator/1  "u1"
  Demux/1 -> Integrator/2  "v0"
  Integrator/1 -> v5/1, Integrator1/1  "v"
  Demux/2 -> Integrator1/2  "p0"
  Integrator1/1 -> p5/1  "p"

== system Experiment1_model/Robots Dynamics Decentralized/Robot6 ==
  In1 : Inport
  Demux : Demux  Outputs=2
  Integrator : Integrator  InitialConditionSource=external  LimitOutput=on  UpperSaturationLimit=2  LowerSaturationLimit=-2
  Integrator1 : Integrator  InitialConditionSource=external
  initial conditions : Constant  Value=[0;0;8;8]  VectorParams1D=off
  p6 : Outport
  v6 : Outport  Port=2
  wires:
  initial conditions/1 -> Demux/1
  In1/1 -> Integrator/1  "u1"
  Demux/1 -> Integrator/2  "v0"
  Integrator/1 -> v6/1, Integrator1/1  "v"
  Demux/2 -> Integrator1/2  "p0"
  Integrator1/1 -> p6/1  "p"

== system Experiment1_model/Robots Dynamics Decentralized/Robot7 ==
  In1 : Inport
  Demux : Demux  Outputs=2
  Integrator : Integrator  InitialConditionSource=external  LimitOutput=on  UpperSaturationLimit=2  LowerSaturationLimit=-2
  Integrator1 : Integrator  InitialConditionSource=external
  initial conditions : Constant  Value=[0;0;10;-10]  VectorParams1D=off
  p7 : Outport
  v7 : Outport  Port=2
  wires:
  initial conditions/1 -> Demux/1
  In1/1 -> Integrator/1  "u1"
  Demux/1 -> Integrator/2  "v0"
  Integrator/1 -> v7/1, Integrator1/1  "v"
  Demux/2 -> Integrator1/2  "p0"
  Integrator1/1 -> p7/1  "p"

== system Experiment1_model/Robots Dynamics Decentralized/Robot8 ==
  In1 : Inport
  Demux : Demux  Outputs=2
  Integrator : Integrator  InitialConditionSource=external  LimitOutput=on  UpperSaturationLimit=2  LowerSaturationLimit=-2
  Integrator1 : Integrator  InitialConditionSource=external
  initial conditions : Constant  Value=[0;0;12;-3]  VectorParams1D=off
  p8 : Outport
  v8 : Outport  Port=2
  wires:
  initial conditions/1 -> Demux/1
  In1/1 -> Integrator/1  "u1"
  Demux/1 -> Integrator/2  "v0"
  Integrator/1 -> v8/1, Integrator1/1  "v"
  Demux/2 -> Integrator1/2  "p0"
  Integrator1/1 -> p8/1  "p"

== system Experiment1_model/Robots Dynamics Decentralized/Visualization ==
  p : Inport
  MATLAB Function : MATLAB Function  TreatAsAtomicUnit=on
  wires:
  p/1 -> MATLAB Function/1(p)

== system Experiment1_model/Robots Dynamics Decentralized/Visualization1 ==
  p : Inport
  MATLAB Function : MATLAB Function  TreatAsAtomicUnit=on
  wires:
  p/1 -> MATLAB Function/1(p)

== system Experiment1_model/Robots Dynamics Decentralized1/Robot1 ==
  In1 : Inport
  Demux : Demux  Outputs=2
  Integrator : Integrator  InitialConditionSource=external  LimitOutput=on  UpperSaturationLimit=2  LowerSaturationLimit=-2
  Integrator1 : Integrator  InitialConditionSource=external
  initial conditions : Constant  Value=[0;0;-10;0]  VectorParams1D=off
  p1 : Outport
  v1 : Outport  Port=2
  wires:
  initial conditions/1 -> Demux/1
  In1/1 -> Integrator/1  "u1"
  Demux/1 -> Integrator/2  "v0"
  Integrator/1 -> Integrator1/1, v1/1  "v"
  Demux/2 -> Integrator1/2  "p0"
  Integrator1/1 -> p1/1  "p"
